simulink library "Byte_Demultiplexers_Lib"  (Simulink 8.7)
settings: Solver=ode45  StartTime=0.0  StopTime=10.0  RelTol=1e-3
libraries: Bit_Demultiplexers_Lib x32, Computer_Library x17, commutil2 x10
settings Model: Creator=uzivatel  LastModifiedBy=Jozko Mrkvicka

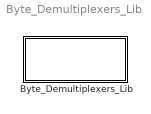
== system Byte_Demultiplexers_Lib ==
  Byte_Demultiplexers_Lib : Subsystem

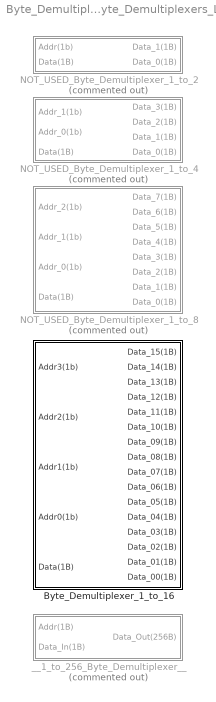
== system Byte_Demultiplexers_Lib/Byte_Demultiplexers_Lib ==
  Byte_Demultiplexer_1_to_16 : Subsystem
  NOT_USED_Byte_Demultiplexer_1_to_2 : Subsystem  Commented=on
  NOT_USED_Byte_Demultiplexer_1_to_4 : Subsystem  Commented=on
  NOT_USED_Byte_Demultiplexer_1_to_8 : Subsystem  Commented=on
  __1_to_256_Byte_Demultiplexer__ : Subsystem  Commented=on

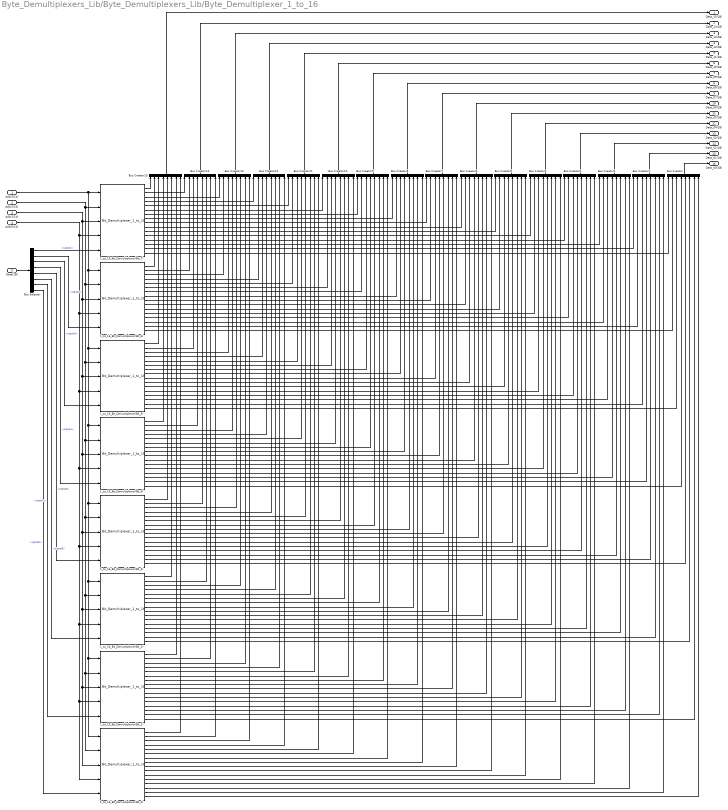
== system Byte_Demultiplexers_Lib/Byte_Demultiplexers_Lib/Byte_Demultiplexer_1_to_16 ==
  Addr3(1b) : Inport
  Addr2(1b) : Inport  Port=2
  Addr1(1b) : Inport  Port=3
  Addr0(1b) : Inport  Port=4
  Data(1B) : Inport  Port=5
  1_to_16_Bit_Demultiplexer(Bit_0) : Bit_Demultiplexers_Lib/Bit_Demultiplexers_Lib/Bit_Demultiplexer_1_to_16
  1_to_16_Bit_Demultiplexer(Bit_1) : Bit_Demultiplexers_Lib/Bit_Demultiplexers_Lib/Bit_Demultiplexer_1_to_16
  1_to_16_Bit_Demultiplexer(Bit_2) : Bit_Demultiplexers_Lib/Bit_Demultiplexers_Lib/Bit_Demultiplexer_1_to_16
  1_to_16_Bit_Demultiplexer(Bit_3) : Bit_Demultiplexers_Lib/Bit_Demultiplexers_Lib/Bit_Demultiplexer_1_to_16
  1_to_16_Bit_Demultiplexer(Bit_4) : Bit_Demultiplexers_Lib/Bit_Demultiplexers_Lib/Bit_Demultiplexer_1_to_16
  1_to_16_Bit_Demultiplexer(Bit_5) : Bit_Demultiplexers_Lib/Bit_Demultiplexers_Lib/Bit_Demultiplexer_1_to_16
  1_to_16_Bit_Demultiplexer(Bit_6) : Bit_Demultiplexers_Lib/Bit_Demultiplexers_Lib/Bit_Demultiplexer_1_to_16
  1_to_16_Bit_Demultiplexer(Bit_7) : Bit_Demultiplexers_Lib/Bit_Demultiplexers_Lib/Bit_Demultiplexer_1_to_16
  Bus Creator{,1..15} (16 alike) : BusCreator  Inputs=8
  Bus Selector : BusSelector  OutputSignals=signal1,signal2,signal3,signal4,signal5,signal6,signal7,signal8
  Data_15(1B) : Outport
  Data_14(1B) : Outport  Port=2
  Data_13(1B) : Outport  Port=3
  Data_12(1B) : Outport  Port=4
  Data_11(1B) : Outport  Port=5
  Data_10(1B) : Outport  Port=6
  Data_09(1B) : Outport  Port=7
  Data_08(1B) : Outport  Port=8
  Data_07(1B) : Outport  Port=9
  Data_06(1B) : Outport  Port=10
  Data_05(1B) : Outport  Port=11
  Data_04(1B) : Outport  Port=12
  Data_03(1B) : Outport  Port=13
  Data_02(1B) : Outport  Port=14
  Data_01(1B) : Outport  Port=15
  Data_00(1B) : Outport  Port=16
  wires:
  Bus Selector/4 -> 1_to_16_Bit_Demultiplexer(Bit_4)/5  "<signal4>"
  Bus Selector/5 -> 1_to_16_Bit_Demultiplexer(Bit_3)/5  "<signal5>"
  Bus Selector/6 -> 1_to_16_Bit_Demultiplexer(Bit_2)/5  "<signal6>"
  Bus Selector/7 -> 1_to_16_Bit_Demultiplexer(Bit_1)/5  "<signal7>"
  Bus Selector/8 -> 1_to_16_Bit_Demultiplexer(Bit_0)/5  "<signal8>"
  Bus Selector/3 -> 1_to_16_Bit_Demultiplexer(Bit_5)/5  "<signal3>"
  Bus Selector/2 -> 1_to_16_Bit_Demultiplexer(Bit_6)/5  "<signal2>"
  Bus Selector/1 -> 1_to_16_Bit_Demultiplexer(Bit_7)/5  "<signal1>"
  Bus Creator15/1 -> Data_15(1B)/1
  Bus Creator14/1 -> Data_14(1B)/1
  Bus Creator13/1 -> Data_13(1B)/1
  Bus Creator12/1 -> Data_12(1B)/1
  Bus Creator11/1 -> Data_11(1B)/1
  Bus Creator10/1 -> Data_10(1B)/1
  Bus Creator9/1 -> Data_09(1B)/1
  Bus Creator8/1 -> Data_08(1B)/1
  Bus Creator7/1 -> Data_07(1B)/1
  Bus Creator6/1 -> Data_06(1B)/1
  Bus Creator5/1 -> Data_05(1B)/1
  Bus Creator4/1 -> Data_04(1B)/1
  Bus Creator3/1 -> Data_03(1B)/1
  Bus Creator2/1 -> Data_02(1B)/1
  Bus Creator1/1 -> Data_01(1B)/1
  Bus Creator/1 -> Data_00(1B)/1
  1_to_16_Bit_Demultiplexer(Bit_0)/16 -> Bus Creator/8
  1_to_16_Bit_Demultiplexer(Bit_0)/15 -> Bus Creator1/8
  1_to_16_Bit_Demultiplexer(Bit_0)/14 -> Bus Creator2/8
  1_to_16_Bit_Demultiplexer(Bit_0)/13 -> Bus Creator3/8
  1_to_16_Bit_Demultiplexer(Bit_0)/12 -> Bus Creator4/8
  1_to_16_Bit_Demultiplexer(Bit_0)/11 -> Bus Creator5/8
  1_to_16_Bit_Demultiplexer(Bit_0)/10 -> Bus Creator6/8
  1_to_16_Bit_Demultiplexer(Bit_0)/9 -> Bus Creator7/8
  1_to_16_Bit_Demultiplexer(Bit_0)/8 -> Bus Creator8/8
  1_to_16_Bit_Demultiplexer(Bit_0)/7 -> Bus Creator9/8
  1_to_16_Bit_Demultiplexer(Bit_0)/6 -> Bus Creator10/8
  1_to_16_Bit_Demultiplexer(Bit_0)/5 -> Bus Creator11/8
  1_to_16_Bit_Demultiplexer(Bit_0)/4 -> Bus Creator12/8
  1_to_16_Bit_Demultiplexer(Bit_0)/3 -> Bus Creator13/8
  1_to_16_Bit_Demultiplexer(Bit_0)/2 -> Bus Creator14/8
  1_to_16_Bit_Demultiplexer(Bit_0)/1 -> Bus Creator15/8
  1_to_16_Bit_Demultiplexer(Bit_1)/16 -> Bus Creator/7
  1_to_16_Bit_Demultiplexer(Bit_1)/15 -> Bus Creator1/7
  1_to_16_Bit_Demultiplexer(Bit_1)/14 -> Bus Creator2/7
  1_to_16_Bit_Demultiplexer(Bit_1)/13 -> Bus Creator3/7
  1_to_16_Bit_Demultiplexer(Bit_1)/12 -> Bus Creator4/7
  1_to_16_Bit_Demultiplexer(Bit_1)/11 -> Bus Creator5/7
  1_to_16_Bit_Demultiplexer(Bit_1)/10 -> Bus Creator6/7
  1_to_16_Bit_Demultiplexer(Bit_1)/9 -> Bus Creator7/7
  1_to_16_Bit_Demultiplexer(Bit_1)/8 -> Bus Creator8/7
  1_to_16_Bit_Demultiplexer(Bit_1)/7 -> Bus Creator9/7
  1_to_16_Bit_Demultiplexer(Bit_1)/6 -> Bus Creator10/7
  1_to_16_Bit_Demultiplexer(Bit_1)/5 -> Bus Creator11/7
  1_to_16_Bit_Demultiplexer(Bit_1)/4 -> Bus Creator12/7
  1_to_16_Bit_Demultiplexer(Bit_1)/3 -> Bus Creator13/7
  1_to_16_Bit_Demultiplexer(Bit_1)/2 -> Bus Creator14/7
  1_to_16_Bit_Demultiplexer(Bit_1)/1 -> Bus Creator15/7
  1_to_16_Bit_Demultiplexer(Bit_2)/16 -> Bus Creator/6
  1_to_16_Bit_Demultiplexer(Bit_2)/15 -> Bus Creator1/6
  1_to_16_Bit_Demultiplexer(Bit_2)/14 -> Bus Creator2/6
  1_to_16_Bit_Demultiplexer(Bit_2)/13 -> Bus Creator3/6
  1_to_16_Bit_Demultiplexer(Bit_2)/12 -> Bus Creator4/6
  1_to_16_Bit_Demultiplexer(Bit_2)/11 -> Bus Creator5/6
  1_to_16_Bit_Demultiplexer(Bit_2)/10 -> Bus Creator6/6
  1_to_16_Bit_Demultiplexer(Bit_2)/9 -> Bus Creator7/6
  1_to_16_Bit_Demultiplexer(Bit_2)/8 -> Bus Creator8/6
  1_to_16_Bit_Demultiplexer(Bit_2)/7 -> Bus Creator9/6
  1_to_16_Bit_Demultiplexer(Bit_2)/6 -> Bus Creator10/6
  1_to_16_Bit_Demultiplexer(Bit_2)/5 -> Bus Creator11/6
  1_to_16_Bit_Demultiplexer(Bit_2)/4 -> Bus Creator12/6
  1_to_16_Bit_Demultiplexer(Bit_2)/3 -> Bus Creator13/6
  1_to_16_Bit_Demultiplexer(Bit_2)/2 -> Bus Creator14/6
  1_to_16_Bit_Demultiplexer(Bit_2)/1 -> Bus Creator15/6
  1_to_16_Bit_Demultiplexer(Bit_3)/16 -> Bus Creator/5
  1_to_16_Bit_Demultiplexer(Bit_3)/15 -> Bus Creator1/5
  1_to_16_Bit_Demultiplexer(Bit_3)/14 -> Bus Creator2/5
  1_to_16_Bit_Demultiplexer(Bit_3)/13 -> Bus Creator3/5
  1_to_16_Bit_Demultiplexer(Bit_3)/12 -> Bus Creator4/5
  1_to_16_Bit_Demultiplexer(Bit_3)/11 -> Bus Creator5/5
  1_to_16_Bit_Demultiplexer(Bit_3)/10 -> Bus Creator6/5
  1_to_16_Bit_Demultiplexer(Bit_3)/9 -> Bus Creator7/5
  1_to_16_Bit_Demultiplexer(Bit_3)/8 -> Bus Creator8/5
  1_to_16_Bit_Demultiplexer(Bit_3)/7 -> Bus Creator9/5
  1_to_16_Bit_Demultiplexer(Bit_3)/6 -> Bus Creator10/5
  1_to_16_Bit_Demultiplexer(Bit_3)/5 -> Bus Creator11/5
  1_to_16_Bit_Demultiplexer(Bit_3)/4 -> Bus Creator12/5
  1_to_16_Bit_Demultiplexer(Bit_3)/3 -> Bus Creator13/5
  1_to_16_Bit_Demultiplexer(Bit_3)/2 -> Bus Creator14/5
  1_to_16_Bit_Demultiplexer(Bit_3)/1 -> Bus Creator15/5
  1_to_16_Bit_Demultiplexer(Bit_4)/16 -> Bus Creator/4
  1_to_16_Bit_Demultiplexer(Bit_4)/15 -> Bus Creator1/4
  1_to_16_Bit_Demultiplexer(Bit_4)/14 -> Bus Creator2/4
  1_to_16_Bit_Demultiplexer(Bit_4)/13 -> Bus Creator3/4
  1_to_16_Bit_Demultiplexer(Bit_4)/12 -> Bus Creator4/4
  1_to_16_Bit_Demultiplexer(Bit_4)/11 -> Bus Creator5/4
  1_to_16_Bit_Demultiplexer(Bit_4)/10 -> Bus Creator6/4
  1_to_16_Bit_Demultiplexer(Bit_4)/9 -> Bus Creator7/4
  1_to_16_Bit_Demultiplexer(Bit_4)/8 -> Bus Creator8/4
  1_to_16_Bit_Demultiplexer(Bit_4)/7 -> Bus Creator9/4
  1_to_16_Bit_Demultiplexer(Bit_4)/6 -> Bus Creator10/4
  1_to_16_Bit_Demultiplexer(Bit_4)/5 -> Bus Creator11/4
  1_to_16_Bit_Demultiplexer(Bit_4)/4 -> Bus Creator12/4
  1_to_16_Bit_Demultiplexer(Bit_4)/3 -> Bus Creator13/4
  1_to_16_Bit_Demultiplexer(Bit_4)/2 -> Bus Creator14/4
  1_to_16_Bit_Demultiplexer(Bit_4)/1 -> Bus Creator15/4
  1_to_16_Bit_Demultiplexer(Bit_5)/16 -> Bus Creator/3
  1_to_16_Bit_Demultiplexer(Bit_5)/15 -> Bus Creator1/3
  1_to_16_Bit_Demultiplexer(Bit_5)/14 -> Bus Creator2/3
  1_to_16_Bit_Demultiplexer(Bit_5)/13 -> Bus Creator3/3
  1_to_16_Bit_Demultiplexer(Bit_5)/12 -> Bus Creator4/3
  1_to_16_Bit_Demultiplexer(Bit_5)/11 -> Bus Creator5/3
  1_to_16_Bit_Demultiplexer(Bit_5)/10 -> Bus Creator6/3
  1_to_16_Bit_Demultiplexer(Bit_5)/9 -> Bus Creator7/3
  1_to_16_Bit_Demultiplexer(Bit_5)/8 -> Bus Creator8/3
  1_to_16_Bit_Demultiplexer(Bit_5)/7 -> Bus Creator9/3
  1_to_16_Bit_Demultiplexer(Bit_5)/6 -> Bus Creator10/3
  1_to_16_Bit_Demultiplexer(Bit_5)/5 -> Bus Creator11/3
  1_to_16_Bit_Demultiplexer(Bit_5)/4 -> Bus Creator12/3
  1_to_16_Bit_Demultiplexer(Bit_5)/3 -> Bus Creator13/3
  1_to_16_Bit_Demultiplexer(Bit_5)/2 -> Bus Creator14/3
  1_to_16_Bit_Demultiplexer(Bit_5)/1 -> Bus Creator15/3
  1_to_16_Bit_Demultiplexer(Bit_6)/16 -> Bus Creator/2
  1_to_16_Bit_Demultiplexer(Bit_6)/15 -> Bus Creator1/2
  1_to_16_Bit_Demultiplexer(Bit_6)/14 -> Bus Creator2/2
  1_to_16_Bit_Demultiplexer(Bit_6)/13 -> Bus Creator3/2
  1_to_16_Bit_Demultiplexer(Bit_6)/12 -> Bus Creator4/2
  1_to_16_Bit_Demultiplexer(Bit_6)/11 -> Bus Creator5/2
  1_to_16_Bit_Demultiplexer(Bit_6)/10 -> Bus Creator6/2
  1_to_16_Bit_Demultiplexer(Bit_6)/9 -> Bus Creator7/2
  1_to_16_Bit_Demultiplexer(Bit_6)/8 -> Bus Creator8/2
  1_to_16_Bit_Demultiplexer(Bit_6)/7 -> Bus Creator9/2
  1_to_16_Bit_Demultiplexer(Bit_6)/6 -> Bus Creator10/2
  1_to_16_Bit_Demultiplexer(Bit_6)/5 -> Bus Creator11/2
  1_to_16_Bit_Demultiplexer(Bit_6)/4 -> Bus Creator12/2
  1_to_16_Bit_Demultiplexer(Bit_6)/3 -> Bus Creator13/2
  1_to_16_Bit_Demultiplexer(Bit_6)/2 -> Bus Creator14/2
  1_to_16_Bit_Demultiplexer(Bit_6)/1 -> Bus Creator15/2
  1_to_16_Bit_Demultiplexer(Bit_7)/16 -> Bus Creator/1
  1_to_16_Bit_Demultiplexer(Bit_7)/15 -> Bus Creator1/1
  1_to_16_Bit_Demultiplexer(Bit_7)/14 -> Bus Creator2/1
  1_to_16_Bit_Demultiplexer(Bit_7)/13 -> Bus Creator3/1
  1_to_16_Bit_Demultiplexer(Bit_7)/12 -> Bus Creator4/1
  1_to_16_Bit_Demultiplexer(Bit_7)/11 -> Bus Creator5/1
  1_to_16_Bit_Demultiplexer(Bit_7)/10 -> Bus Creator6/1
  1_to_16_Bit_Demultiplexer(Bit_7)/9 -> Bus Creator7/1
  1_to_16_Bit_Demultiplexer(Bit_7)/8 -> Bus Creator8/1
  1_to_16_Bit_Demultiplexer(Bit_7)/7 -> Bus Creator9/1
  1_to_16_Bit_Demultiplexer(Bit_7)/6 -> Bus Creator10/1
  1_to_16_Bit_Demultiplexer(Bit_7)/5 -> Bus Creator11/1
  1_to_16_Bit_Demultiplexer(Bit_7)/4 -> Bus Creator12/1
  1_to_16_Bit_Demultiplexer(Bit_7)/3 -> Bus Creator13/1
  1_to_16_Bit_Demultiplexer(Bit_7)/2 -> Bus Creator14/1
  1_to_16_Bit_Demultiplexer(Bit_7)/1 -> Bus Creator15/1
  Data(1B)/1 -> Bus Selector/1
  Addr3(1b)/1 -> 1_to_16_Bit_Demultiplexer(Bit_7)/1, 1_to_16_Bit_Demultiplexer(Bit_6)/1, 1_to_16_Bit_Demultiplexer(Bit_5)/1, 1_to_16_Bit_Demultiplexer(Bit_4)/1, 1_to_16_Bit_Demultiplexer(Bit_3)/1, 1_to_16_Bit_Demultiplexer(Bit_2)/1, 1_to_16_Bit_Demultiplexer(Bit_1)/1, 1_to_16_Bit_Demultiplexer(Bit_0)/1
  Addr2(1b)/1 -> 1_to_16_Bit_Demultiplexer(Bit_6)/2, 1_to_16_Bit_Demultiplexer(Bit_5)/2, 1_to_16_Bit_Demultiplexer(Bit_4)/2, 1_to_16_Bit_Demultiplexer(Bit_3)/2, 1_to_16_Bit_Demultiplexer(Bit_2)/2, 1_to_16_Bit_Demultiplexer(Bit_1)/2, 1_to_16_Bit_Demultiplexer(Bit_0)/2, 1_to_16_Bit_Demultiplexer(Bit_7)/2
  Addr1(1b)/1 -> 1_to_16_Bit_Demultiplexer(Bit_6)/3, 1_to_16_Bit_Demultiplexer(Bit_5)/3, 1_to_16_Bit_Demultiplexer(Bit_4)/3, 1_to_16_Bit_Demultiplexer(Bit_3)/3, 1_to_16_Bit_Demultiplexer(Bit_2)/3, 1_to_16_Bit_Demultiplexer(Bit_1)/3, 1_to_16_Bit_Demultiplexer(Bit_0)/3, 1_to_16_Bit_Demultiplexer(Bit_7)/3
  Addr0(1b)/1 -> 1_to_16_Bit_Demultiplexer(Bit_6)/4, 1_to_16_Bit_Demultiplexer(Bit_5)/4, 1_to_16_Bit_Demultiplexer(Bit_4)/4, 1_to_16_Bit_Demultiplexer(Bit_3)/4, 1_to_16_Bit_Demultiplexer(Bit_2)/4, 1_to_16_Bit_Demultiplexer(Bit_0)/4, 1_to_16_Bit_Demultiplexer(Bit_1)/4, 1_to_16_Bit_Demultiplexer(Bit_7)/4

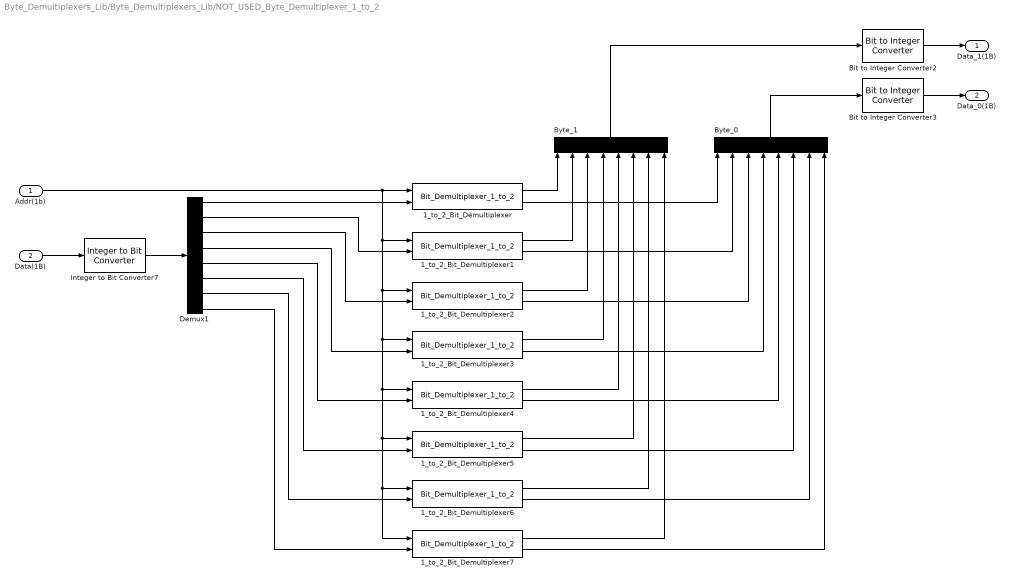
== system Byte_Demultiplexers_Lib/Byte_Demultiplexers_Lib/NOT_USED_Byte_Demultiplexer_1_to_2 ==
  Addr(1b) : Inport
  Data(1B) : Inport  Port=2
  1_to_2_Bit_Demultiplexer{,1..7} (8 alike) : Bit_Demultiplexers_Lib/Bit_Demultiplexers_Lib/Bit_Demultiplexer_1_to_2
  Bit to Integer Converter2 : commutil2/Bit to Integer Converter  nbits=8  bitOrder=MSB first  signedOutputValues=Unsigned  outDtype=uint8  outDtypeSigned=Inherit via internal rule
  Bit to Integer Converter3 : commutil2/Bit to Integer Converter  nbits=8  bitOrder=MSB first  signedOutputValues=Unsigned  outDtype=uint8  outDtypeSigned=Inherit via internal rule
  Byte_0 : Mux  Inputs=8
  Byte_1 : Mux  Inputs=8
  Demux1 : Demux  Outputs=8
  Integer to Bit Converter7 : commutil2/Integer to Bit Converter  nbits=8  signedInputValues=Unsigned  bitOrder=MSB first  outDtype=boolean
  Data_1(1B) : Outport
  Data_0(1B) : Outport  Port=2
  wires:
  Demux1/4 -> 1_to_2_Bit_Demultiplexer3/2
  Demux1/5 -> 1_to_2_Bit_Demultiplexer4/2
  Demux1/6 -> 1_to_2_Bit_Demultiplexer5/2
  Demux1/7 -> 1_to_2_Bit_Demultiplexer6/2
  Demux1/8 -> 1_to_2_Bit_Demultiplexer7/2
  Demux1/3 -> 1_to_2_Bit_Demultiplexer2/2
  Demux1/2 -> 1_to_2_Bit_Demultiplexer1/2
  Demux1/1 -> 1_to_2_Bit_Demultiplexer/2
  Byte_1/1 -> Bit to Integer Converter2/1
  Byte_0/1 -> Bit to Integer Converter3/1
  1_to_2_Bit_Demultiplexer7/2 -> Byte_0/8
  1_to_2_Bit_Demultiplexer7/1 -> Byte_1/8
  1_to_2_Bit_Demultiplexer6/2 -> Byte_0/7
  1_to_2_Bit_Demultiplexer6/1 -> Byte_1/7
  1_to_2_Bit_Demultiplexer5/2 -> Byte_0/6
  1_to_2_Bit_Demultiplexer5/1 -> Byte_1/6
  1_to_2_Bit_Demultiplexer4/2 -> Byte_0/5
  1_to_2_Bit_Demultiplexer4/1 -> Byte_1/5
  1_to_2_Bit_Demultiplexer3/2 -> Byte_0/4
  1_to_2_Bit_Demultiplexer3/1 -> Byte_1/4
  1_to_2_Bit_Demultiplexer2/2 -> Byte_0/3
  1_to_2_Bit_Demultiplexer2/1 -> Byte_1/3
  1_to_2_Bit_Demultiplexer1/2 -> Byte_0/2
  1_to_2_Bit_Demultiplexer1/1 -> Byte_1/2
  1_to_2_Bit_Demultiplexer/2 -> Byte_0/1
  1_to_2_Bit_Demultiplexer/1 -> Byte_1/1
  Integer to Bit Converter7/1 -> Demux1/1
  Data(1B)/1 -> Integer to Bit Converter7/1
  Addr(1b)/1 -> 1_to_2_Bit_Demultiplexer/1, 1_to_2_Bit_Demultiplexer7/1, 1_to_2_Bit_Demultiplexer6/1, 1_to_2_Bit_Demultiplexer5/1, 1_to_2_Bit_Demultiplexer4/1, 1_to_2_Bit_Demultiplexer3/1, 1_to_2_Bit_Demultiplexer2/1, 1_to_2_Bit_Demultiplexer1/1
  Bit to Integer Converter2/1 -> Data_1(1B)/1
  Bit to Integer Converter3/1 -> Data_0(1B)/1

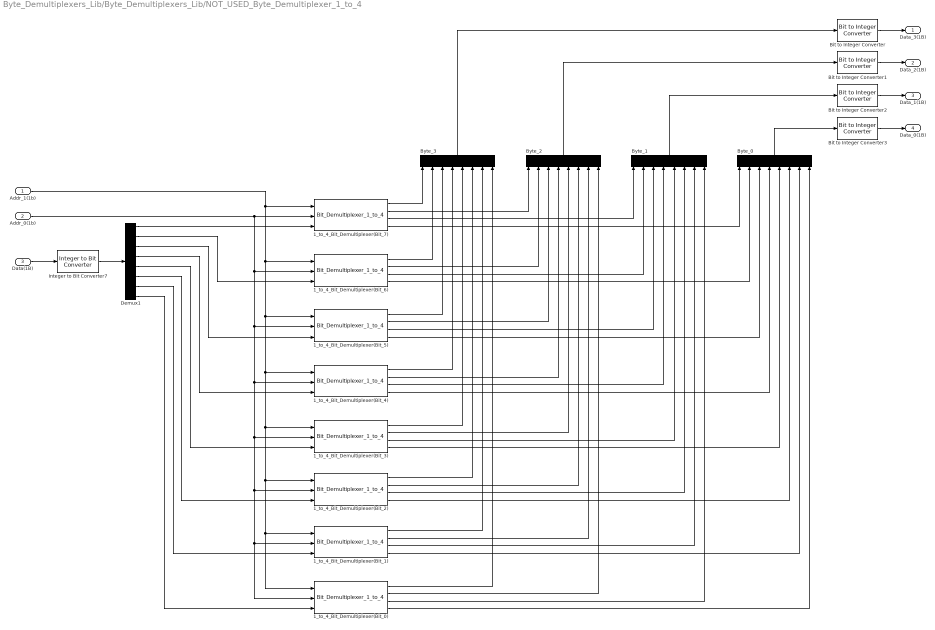
== system Byte_Demultiplexers_Lib/Byte_Demultiplexers_Lib/NOT_USED_Byte_Demultiplexer_1_to_4 ==
  Addr_1(1b) : Inport
  Addr_0(1b) : Inport  Port=2
  Data(1B) : Inport  Port=3
  1_to_4_Bit_Demultiplexer(Bit_0) : Bit_Demultiplexers_Lib/Bit_Demultiplexers_Lib/Bit_Demultiplexer_1_to_4
  1_to_4_Bit_Demultiplexer(Bit_1) : Bit_Demultiplexers_Lib/Bit_Demultiplexers_Lib/Bit_Demultiplexer_1_to_4
  1_to_4_Bit_Demultiplexer(Bit_2) : Bit_Demultiplexers_Lib/Bit_Demultiplexers_Lib/Bit_Demultiplexer_1_to_4
  1_to_4_Bit_Demultiplexer(Bit_3) : Bit_Demultiplexers_Lib/Bit_Demultiplexers_Lib/Bit_Demultiplexer_1_to_4
  1_to_4_Bit_Demultiplexer(Bit_4) : Bit_Demultiplexers_Lib/Bit_Demultiplexers_Lib/Bit_Demultiplexer_1_to_4
  1_to_4_Bit_Demultiplexer(Bit_5) : Bit_Demultiplexers_Lib/Bit_Demultiplexers_Lib/Bit_Demultiplexer_1_to_4
  1_to_4_Bit_Demultiplexer(Bit_6) : Bit_Demultiplexers_Lib/Bit_Demultiplexers_Lib/Bit_Demultiplexer_1_to_4
  1_to_4_Bit_Demultiplexer(Bit_7) : Bit_Demultiplexers_Lib/Bit_Demultiplexers_Lib/Bit_Demultiplexer_1_to_4
  Bit to Integer Converter{,1..3} (4 alike) : commutil2/Bit to Integer Converter  nbits=8  bitOrder=MSB first  signedOutputValues=Unsigned  outDtype=uint8  outDtypeSigned=Inherit via internal rule
  Byte_{0..3} (4 alike) : Mux  Inputs=8
  Demux1 : Demux  Outputs=8
  Integer to Bit Converter7 : commutil2/Integer to Bit Converter  nbits=8  signedInputValues=Unsigned  bitOrder=MSB first  outDtype=boolean
  Data_3(1B) : Outport
  Data_2(1B) : Outport  Port=2
  Data_1(1B) : Outport  Port=3
  Data_0(1B) : Outport  Port=4
  wires:
  Bit to Integer Converter/1 -> Data_3(1B)/1
  Demux1/4 -> 1_to_4_Bit_Demultiplexer(Bit_4)/3
  Demux1/5 -> 1_to_4_Bit_Demultiplexer(Bit_3)/3
  Demux1/6 -> 1_to_4_Bit_Demultiplexer(Bit_2)/3
  Demux1/7 -> 1_to_4_Bit_Demultiplexer(Bit_1)/3
  Demux1/8 -> 1_to_4_Bit_Demultiplexer(Bit_0)/3
  Demux1/3 -> 1_to_4_Bit_Demultiplexer(Bit_5)/3
  Demux1/2 -> 1_to_4_Bit_Demultiplexer(Bit_6)/3
  Demux1/1 -> 1_to_4_Bit_Demultiplexer(Bit_7)/3
  Byte_3/1 -> Bit to Integer Converter/1
  Byte_2/1 -> Bit to Integer Converter1/1
  Byte_1/1 -> Bit to Integer Converter2/1
  Byte_0/1 -> Bit to Integer Converter3/1
  1_to_4_Bit_Demultiplexer(Bit_0)/4 -> Byte_0/8
  1_to_4_Bit_Demultiplexer(Bit_0)/3 -> Byte_1/8
  1_to_4_Bit_Demultiplexer(Bit_0)/2 -> Byte_2/8
  1_to_4_Bit_Demultiplexer(Bit_0)/1 -> Byte_3/8
  1_to_4_Bit_Demultiplexer(Bit_1)/4 -> Byte_0/7
  1_to_4_Bit_Demultiplexer(Bit_1)/3 -> Byte_1/7
  1_to_4_Bit_Demultiplexer(Bit_1)/2 -> Byte_2/7
  1_to_4_Bit_Demultiplexer(Bit_1)/1 -> Byte_3/7
  1_to_4_Bit_Demultiplexer(Bit_2)/4 -> Byte_0/6
  1_to_4_Bit_Demultiplexer(Bit_2)/3 -> Byte_1/6
  1_to_4_Bit_Demultiplexer(Bit_2)/2 -> Byte_2/6
  1_to_4_Bit_Demultiplexer(Bit_2)/1 -> Byte_3/6
  1_to_4_Bit_Demultiplexer(Bit_3)/4 -> Byte_0/5
  1_to_4_Bit_Demultiplexer(Bit_3)/3 -> Byte_1/5
  1_to_4_Bit_Demultiplexer(Bit_3)/2 -> Byte_2/5
  1_to_4_Bit_Demultiplexer(Bit_3)/1 -> Byte_3/5
  1_to_4_Bit_Demultiplexer(Bit_4)/4 -> Byte_0/4
  1_to_4_Bit_Demultiplexer(Bit_4)/3 -> Byte_1/4
  1_to_4_Bit_Demultiplexer(Bit_4)/2 -> Byte_2/4
  1_to_4_Bit_Demultiplexer(Bit_4)/1 -> Byte_3/4
  1_to_4_Bit_Demultiplexer(Bit_5)/4 -> Byte_0/3
  1_to_4_Bit_Demultiplexer(Bit_5)/3 -> Byte_1/3
  1_to_4_Bit_Demultiplexer(Bit_5)/2 -> Byte_2/3
  1_to_4_Bit_Demultiplexer(Bit_5)/1 -> Byte_3/3
  1_to_4_Bit_Demultiplexer(Bit_6)/4 -> Byte_0/2
  1_to_4_Bit_Demultiplexer(Bit_6)/3 -> Byte_1/2
  1_to_4_Bit_Demultiplexer(Bit_6)/2 -> Byte_2/2
  1_to_4_Bit_Demultiplexer(Bit_6)/1 -> Byte_3/2
  1_to_4_Bit_Demultiplexer(Bit_7)/4 -> Byte_0/1
  1_to_4_Bit_Demultiplexer(Bit_7)/3 -> Byte_1/1
  1_to_4_Bit_Demultiplexer(Bit_7)/2 -> Byte_2/1
  1_to_4_Bit_Demultiplexer(Bit_7)/1 -> Byte_3/1
  Integer to Bit Converter7/1 -> Demux1/1
  Data(1B)/1 -> Integer to Bit Converter7/1
  Addr_0(1b)/1 -> 1_to_4_Bit_Demultiplexer(Bit_7)/2, 1_to_4_Bit_Demultiplexer(Bit_3)/2, 1_to_4_Bit_Demultiplexer(Bit_2)/2, 1_to_4_Bit_Demultiplexer(Bit_1)/2, 1_to_4_Bit_Demultiplexer(Bit_0)/2, 1_to_4_Bit_Demultiplexer(Bit_4)/2, 1_to_4_Bit_Demultiplexer(Bit_5)/2, 1_to_4_Bit_Demultiplexer(Bit_6)/2
  Addr_1(1b)/1 -> 1_to_4_Bit_Demultiplexer(Bit_7)/1, 1_to_4_Bit_Demultiplexer(Bit_0)/1, 1_to_4_Bit_Demultiplexer(Bit_1)/1, 1_to_4_Bit_Demultiplexer(Bit_2)/1, 1_to_4_Bit_Demultiplexer(Bit_3)/1, 1_to_4_Bit_Demultiplexer(Bit_4)/1, 1_to_4_Bit_Demultiplexer(Bit_5)/1, 1_to_4_Bit_Demultiplexer(Bit_6)/1
  Bit to Integer Converter1/1 -> Data_2(1B)/1
  Bit to Integer Converter2/1 -> Data_1(1B)/1
  Bit to Integer Converter3/1 -> Data_0(1B)/1

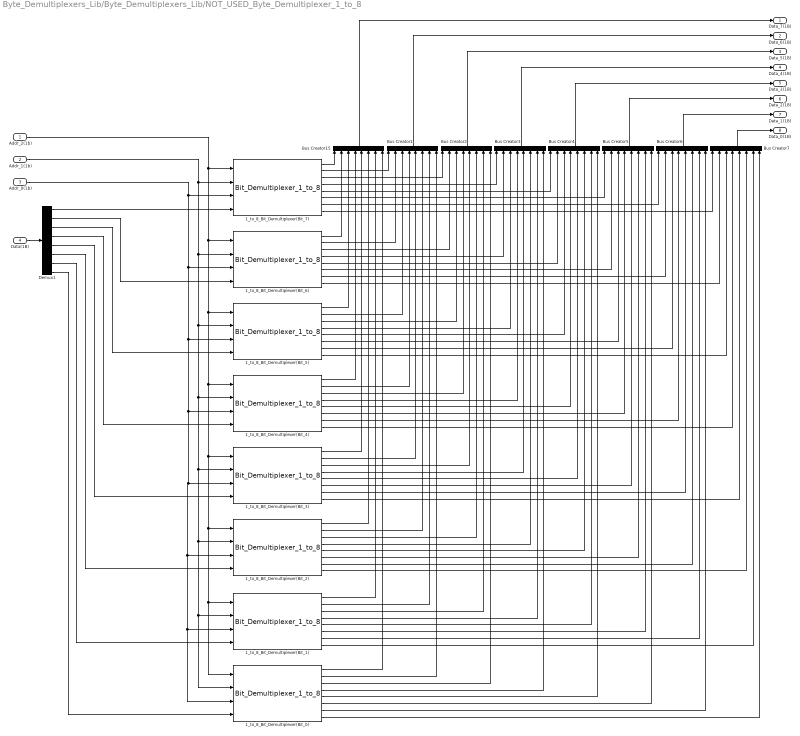
== system Byte_Demultiplexers_Lib/Byte_Demultiplexers_Lib/NOT_USED_Byte_Demultiplexer_1_to_8 ==
  Addr_2(1b) : Inport
  Addr_1(1b) : Inport  Port=2
  Addr_0(1b) : Inport  Port=3
  Data(1B) : Inport  Port=4
  1_to_8_Bit_Demultiplexer(Bit_0) : Bit_Demultiplexers_Lib/Bit_Demultiplexers_Lib/Bit_Demultiplexer_1_to_8
  1_to_8_Bit_Demultiplexer(Bit_1) : Bit_Demultiplexers_Lib/Bit_Demultiplexers_Lib/Bit_Demultiplexer_1_to_8
  1_to_8_Bit_Demultiplexer(Bit_2) : Bit_Demultiplexers_Lib/Bit_Demultiplexers_Lib/Bit_Demultiplexer_1_to_8
  1_to_8_Bit_Demultiplexer(Bit_3) : Bit_Demultiplexers_Lib/Bit_Demultiplexers_Lib/Bit_Demultiplexer_1_to_8
  1_to_8_Bit_Demultiplexer(Bit_4) : Bit_Demultiplexers_Lib/Bit_Demultiplexers_Lib/Bit_Demultiplexer_1_to_8
  1_to_8_Bit_Demultiplexer(Bit_5) : Bit_Demultiplexers_Lib/Bit_Demultiplexers_Lib/Bit_Demultiplexer_1_to_8
  1_to_8_Bit_Demultiplexer(Bit_6) : Bit_Demultiplexers_Lib/Bit_Demultiplexers_Lib/Bit_Demultiplexer_1_to_8
  1_to_8_Bit_Demultiplexer(Bit_7) : Bit_Demultiplexers_Lib/Bit_Demultiplexers_Lib/Bit_Demultiplexer_1_to_8
  Bus Creator{1..7,15} (8 alike) : BusCreator  Inputs=8
  Demux1 : Demux  Outputs=8
  Data_7(1B) : Outport
  Data_6(1B) : Outport  Port=2
  Data_5(1B) : Outport  Port=3
  Data_4(1B) : Outport  Port=4
  Data_3(1B) : Outport  Port=5
  Data_2(1B) : Outport  Port=6
  Data_1(1B) : Outport  Port=7
  Data_0(1B) : Outport  Port=8
  wires:
  Demux1/4 -> 1_to_8_Bit_Demultiplexer(Bit_4)/4
  Demux1/5 -> 1_to_8_Bit_Demultiplexer(Bit_3)/4
  Demux1/6 -> 1_to_8_Bit_Demultiplexer(Bit_2)/4
  Demux1/7 -> 1_to_8_Bit_Demultiplexer(Bit_1)/4
  Demux1/8 -> 1_to_8_Bit_Demultiplexer(Bit_0)/4
  Demux1/3 -> 1_to_8_Bit_Demultiplexer(Bit_5)/4
  Demux1/2 -> 1_to_8_Bit_Demultiplexer(Bit_6)/4
  Demux1/1 -> 1_to_8_Bit_Demultiplexer(Bit_7)/4
  1_to_8_Bit_Demultiplexer(Bit_0)/8 -> Bus Creator7/8
  1_to_8_Bit_Demultiplexer(Bit_0)/7 -> Bus Creator6/8
  1_to_8_Bit_Demultiplexer(Bit_0)/6 -> Bus Creator5/8
  1_to_8_Bit_Demultiplexer(Bit_0)/5 -> Bus Creator4/8
  1_to_8_Bit_Demultiplexer(Bit_0)/4 -> Bus Creator3/8
  1_to_8_Bit_Demultiplexer(Bit_0)/3 -> Bus Creator2/8
  1_to_8_Bit_Demultiplexer(Bit_0)/2 -> Bus Creator1/8
  1_to_8_Bit_Demultiplexer(Bit_0)/1 -> Bus Creator15/8
  1_to_8_Bit_Demultiplexer(Bit_1)/8 -> Bus Creator7/7
  1_to_8_Bit_Demultiplexer(Bit_1)/7 -> Bus Creator6/7
  1_to_8_Bit_Demultiplexer(Bit_1)/6 -> Bus Creator5/7
  1_to_8_Bit_Demultiplexer(Bit_1)/5 -> Bus Creator4/7
  1_to_8_Bit_Demultiplexer(Bit_1)/4 -> Bus Creator3/7
  1_to_8_Bit_Demultiplexer(Bit_1)/3 -> Bus Creator2/7
  1_to_8_Bit_Demultiplexer(Bit_1)/2 -> Bus Creator1/7
  1_to_8_Bit_Demultiplexer(Bit_1)/1 -> Bus Creator15/7
  1_to_8_Bit_Demultiplexer(Bit_2)/8 -> Bus Creator7/6
  1_to_8_Bit_Demultiplexer(Bit_2)/7 -> Bus Creator6/6
  1_to_8_Bit_Demultiplexer(Bit_2)/6 -> Bus Creator5/6
  1_to_8_Bit_Demultiplexer(Bit_2)/5 -> Bus Creator4/6
  1_to_8_Bit_Demultiplexer(Bit_2)/4 -> Bus Creator3/6
  1_to_8_Bit_Demultiplexer(Bit_2)/3 -> Bus Creator2/6
  1_to_8_Bit_Demultiplexer(Bit_2)/2 -> Bus Creator1/6
  1_to_8_Bit_Demultiplexer(Bit_2)/1 -> Bus Creator15/6
  1_to_8_Bit_Demultiplexer(Bit_3)/8 -> Bus Creator7/5
  1_to_8_Bit_Demultiplexer(Bit_3)/7 -> Bus Creator6/5
  1_to_8_Bit_Demultiplexer(Bit_3)/6 -> Bus Creator5/5
  1_to_8_Bit_Demultiplexer(Bit_3)/5 -> Bus Creator4/5
  1_to_8_Bit_Demultiplexer(Bit_3)/4 -> Bus Creator3/5
  1_to_8_Bit_Demultiplexer(Bit_3)/3 -> Bus Creator2/5
  1_to_8_Bit_Demultiplexer(Bit_3)/2 -> Bus Creator1/5
  1_to_8_Bit_Demultiplexer(Bit_3)/1 -> Bus Creator15/5
  1_to_8_Bit_Demultiplexer(Bit_4)/8 -> Bus Creator7/4
  1_to_8_Bit_Demultiplexer(Bit_4)/7 -> Bus Creator6/4
  1_to_8_Bit_Demultiplexer(Bit_4)/6 -> Bus Creator5/4
  1_to_8_Bit_Demultiplexer(Bit_4)/5 -> Bus Creator4/4
  1_to_8_Bit_Demultiplexer(Bit_4)/4 -> Bus Creator3/4
  1_to_8_Bit_Demultiplexer(Bit_4)/3 -> Bus Creator2/4
  1_to_8_Bit_Demultiplexer(Bit_4)/2 -> Bus Creator1/4
  1_to_8_Bit_Demultiplexer(Bit_4)/1 -> Bus Creator15/4
  1_to_8_Bit_Demultiplexer(Bit_5)/8 -> Bus Creator7/3
  1_to_8_Bit_Demultiplexer(Bit_5)/7 -> Bus Creator6/3
  1_to_8_Bit_Demultiplexer(Bit_5)/6 -> Bus Creator5/3
  1_to_8_Bit_Demultiplexer(Bit_5)/5 -> Bus Creator4/3
  1_to_8_Bit_Demultiplexer(Bit_5)/4 -> Bus Creator3/3
  1_to_8_Bit_Demultiplexer(Bit_5)/3 -> Bus Creator2/3
  1_to_8_Bit_Demultiplexer(Bit_5)/2 -> Bus Creator1/3
  1_to_8_Bit_Demultiplexer(Bit_5)/1 -> Bus Creator15/3
  1_to_8_Bit_Demultiplexer(Bit_6)/8 -> Bus Creator7/2
  1_to_8_Bit_Demultiplexer(Bit_6)/7 -> Bus Creator6/2
  1_to_8_Bit_Demultiplexer(Bit_6)/6 -> Bus Creator5/2
  1_to_8_Bit_Demultiplexer(Bit_6)/5 -> Bus Creator4/2
  1_to_8_Bit_Demultiplexer(Bit_6)/4 -> Bus Creator3/2
  1_to_8_Bit_Demultiplexer(Bit_6)/3 -> Bus Creator2/2
  1_to_8_Bit_Demultiplexer(Bit_6)/2 -> Bus Creator1/2
  1_to_8_Bit_Demultiplexer(Bit_6)/1 -> Bus Creator15/2
  1_to_8_Bit_Demultiplexer(Bit_7)/8 -> Bus Creator7/1
  1_to_8_Bit_Demultiplexer(Bit_7)/7 -> Bus Creator6/1
  1_to_8_Bit_Demultiplexer(Bit_7)/6 -> Bus Creator5/1
  1_to_8_Bit_Demultiplexer(Bit_7)/5 -> Bus Creator4/1
  1_to_8_Bit_Demultiplexer(Bit_7)/4 -> Bus Creator3/1
  1_to_8_Bit_Demultiplexer(Bit_7)/3 -> Bus Creator2/1
  1_to_8_Bit_Demultiplexer(Bit_7)/2 -> Bus Creator1/1
  1_to_8_Bit_Demultiplexer(Bit_7)/1 -> Bus Creator15/1
  Data(1B)/1 -> Demux1/1
  Addr_0(1b)/1 -> 1_to_8_Bit_Demultiplexer(Bit_7)/3, 1_to_8_Bit_Demultiplexer(Bit_6)/3, 1_to_8_Bit_Demultiplexer(Bit_5)/3, 1_to_8_Bit_Demultiplexer(Bit_0)/3, 1_to_8_Bit_Demultiplexer(Bit_1)/3, 1_to_8_Bit_Demultiplexer(Bit_2)/3, 1_to_8_Bit_Demultiplexer(Bit_3)/3, 1_to_8_Bit_Demultiplexer(Bit_4)/3
  Addr_1(1b)/1 -> 1_to_8_Bit_Demultiplexer(Bit_7)/2, 1_to_8_Bit_Demultiplexer(Bit_0)/2, 1_to_8_Bit_Demultiplexer(Bit_1)/2, 1_to_8_Bit_Demultiplexer(Bit_2)/2, 1_to_8_Bit_Demultiplexer(Bit_3)/2, 1_to_8_Bit_Demultiplexer(Bit_4)/2, 1_to_8_Bit_Demultiplexer(Bit_5)/2, 1_to_8_Bit_Demultiplexer(Bit_6)/2
  Addr_2(1b)/1 -> 1_to_8_Bit_Demultiplexer(Bit_7)/1, 1_to_8_Bit_Demultiplexer(Bit_0)/1, 1_to_8_Bit_Demultiplexer(Bit_1)/1, 1_to_8_Bit_Demultiplexer(Bit_2)/1, 1_to_8_Bit_Demultiplexer(Bit_3)/1, 1_to_8_Bit_Demultiplexer(Bit_4)/1, 1_to_8_Bit_Demultiplexer(Bit_5)/1, 1_to_8_Bit_Demultiplexer(Bit_6)/1
  Bus Creator7/1 -> Data_0(1B)/1
  Bus Creator6/1 -> Data_1(1B)/1
  Bus Creator5/1 -> Data_2(1B)/1
  Bus Creator4/1 -> Data_3(1B)/1
  Bus Creator3/1 -> Data_4(1B)/1
  Bus Creator2/1 -> Data_5(1B)/1
  Bus Creator1/1 -> Data_6(1B)/1
  Bus Creator15/1 -> Data_7(1B)/1

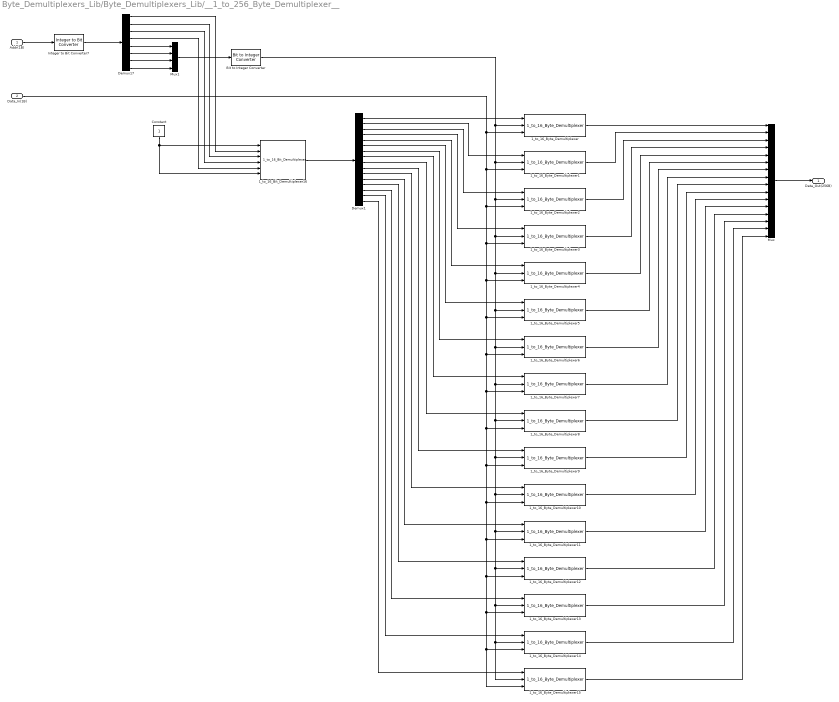
== system Byte_Demultiplexers_Lib/Byte_Demultiplexers_Lib/__1_to_256_Byte_Demultiplexer__ ==
  Addr(1B) : Inport
  Data_In(1B) : Inport  Port=2
  1_to_16_Bit_Demultiplexer16 : Computer_Library/Demultiplexers/1_to_16_Bit_Demultiplexer
  1_to_16_Byte_Demultiplexer{,1..15} (16 alike) : Computer_Library/Demultiplexers/1_to_16_Byte_Demultiplexer
  Bit to Integer Converter : commutil2/Bit to Integer Converter  nbits=4  bitOrder=MSB first  signedOutputValues=Unsigned  outDtype=uint8  outDtypeSigned=Inherit via internal rule
  Constant : Constant
  Demux1 : Demux  Outputs=16
  Demux17 : Demux  Outputs=8
  Integer to Bit Converter7 : commutil2/Integer to Bit Converter  nbits=8  signedInputValues=Unsigned  bitOrder=MSB first  outDtype=boolean
  Mux : Mux  Inputs=16
  Mux1 : Mux
  Data_Out(256B) : Outport  OutDataTypeStr=uint8
  wires:
  Mux1/1 -> Bit to Integer Converter/1
  Addr(1B)/1 -> Integer to Bit Converter7/1
  Integer to Bit Converter7/1 -> Demux17/1
  Bit to Integer Converter/1 -> 1_to_16_Byte_Demultiplexer2/2, 1_to_16_Byte_Demultiplexer3/2, 1_to_16_Byte_Demultiplexer4/2, 1_to_16_Byte_Demultiplexer15/2, 1_to_16_Byte_Demultiplexer14/2, 1_to_16_Byte_Demultiplexer13/2, 1_to_16_Byte_Demultiplexer12/2, 1_to_16_Byte_Demultiplexer11/2, 1_to_16_Byte_Demultiplexer10/2, 1_to_16_Byte_Demultiplexer9/2, 1_to_16_Byte_Demultiplexer8/2, 1_to_16_Byte_Demultiplexer7/2, 1_to_16_Byte_Demultiplexer6/2, 1_to_16_Byte_Demultiplexer5/2, 1_to_16_Byte_Demultiplexer1/2, 1_to_16_Byte_Demultiplexer/2
  Demux17/8 -> Mux1/4
  Demux17/7 -> Mux1/3
  Demux17/6 -> Mux1/2
  Demux17/5 -> Mux1/1
  Demux17/3 -> 1_to_16_Bit_Demultiplexer16/4
  Demux17/4 -> 1_to_16_Bit_Demultiplexer16/5
  Demux17/2 -> 1_to_16_Bit_Demultiplexer16/3
  Demux17/1 -> 1_to_16_Bit_Demultiplexer16/2
  Mux/1 -> Data_Out(256B)/1
  Constant/1 -> 1_to_16_Bit_Demultiplexer16/6, 1_to_16_Bit_Demultiplexer16/1
  Demux1/16 -> 1_to_16_Byte_Demultiplexer15/1
  Demux1/15 -> 1_to_16_Byte_Demultiplexer14/1
  Demux1/14 -> 1_to_16_Byte_Demultiplexer13/1
  Demux1/13 -> 1_to_16_Byte_Demultiplexer12/1
  Demux1/12 -> 1_to_16_Byte_Demultiplexer11/1
  Demux1/11 -> 1_to_16_Byte_Demultiplexer10/1
  Demux1/10 -> 1_to_16_Byte_Demultiplexer9/1
  Demux1/9 -> 1_to_16_Byte_Demultiplexer8/1
  Demux1/8 -> 1_to_16_Byte_Demultiplexer7/1
  Demux1/7 -> 1_to_16_Byte_Demultiplexer6/1
  Demux1/6 -> 1_to_16_Byte_Demultiplexer5/1
  Demux1/5 -> 1_to_16_Byte_Demultiplexer4/1
  Demux1/4 -> 1_to_16_Byte_Demultiplexer3/1
  Demux1/3 -> 1_to_16_Byte_Demultiplexer2/1
  Demux1/2 -> 1_to_16_Byte_Demultiplexer1/1
  Demux1/1 -> 1_to_16_Byte_Demultiplexer/1
  1_to_16_Bit_Demultiplexer16/1 -> Demux1/1
  Data_In(1B)/1 -> 1_to_16_Byte_Demultiplexer/3, 1_to_16_Byte_Demultiplexer1/3, 1_to_16_Byte_Demultiplexer2/3, 1_to_16_Byte_Demultiplexer3/3, 1_to_16_Byte_Demultiplexer4/3, 1_to_16_Byte_Demultiplexer5/3, 1_to_16_Byte_Demultiplexer6/3, 1_to_16_Byte_Demultiplexer7/3, 1_to_16_Byte_Demultiplexer8/3, 1_to_16_Byte_Demultiplexer9/3, 1_to_16_Byte_Demultiplexer10/3, 1_to_16_Byte_Demultiplexer11/3, 1_to_16_Byte_Demultiplexer12/3, 1_to_16_Byte_Demultiplexer13/3, 1_to_16_Byte_Demultiplexer14/3, 1_to_16_Byte_Demultiplexer15/3
  1_to_16_Byte_Demultiplexer/1 -> Mux/1
  1_to_16_Byte_Demultiplexer1/1 -> Mux/2
  1_to_16_Byte_Demultiplexer2/1 -> Mux/3
  1_to_16_Byte_Demultiplexer3/1 -> Mux/4
  1_to_16_Byte_Demultiplexer15/1 -> Mux/16
  1_to_16_Byte_Demultiplexer14/1 -> Mux/15
  1_to_16_Byte_Demultiplexer13/1 -> Mux/14
  1_to_16_Byte_Demultiplexer12/1 -> Mux/13
  1_to_16_Byte_Demultiplexer11/1 -> Mux/12
  1_to_16_Byte_Demultiplexer10/1 -> Mux/11
  1_to_16_Byte_Demultiplexer9/1 -> Mux/10
  1_to_16_Byte_Demultiplexer8/1 -> Mux/9
  1_to_16_Byte_Demultiplexer7/1 -> Mux/8
  1_to_16_Byte_Demultiplexer6/1 -> Mux/7
  1_to_16_Byte_Demultiplexer5/1 -> Mux/6
  1_to_16_Byte_Demultiplexer4/1 -> Mux/5
